simulink subsystem "PieroAJModelz"  (R2023b)
settings: Solver=VariableStepAuto  StartTime=0.0  StopTime=10.0  RelTol=1e-3
settings Model: Creator=Antonio  LastModifiedBy=Antonio

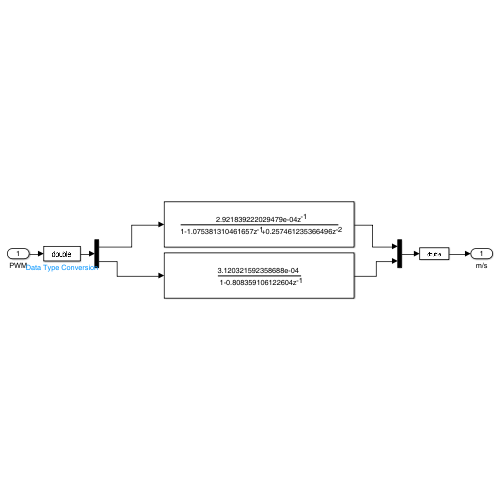
[thumbnail: Simulink's stored preview of the top-level diagram]
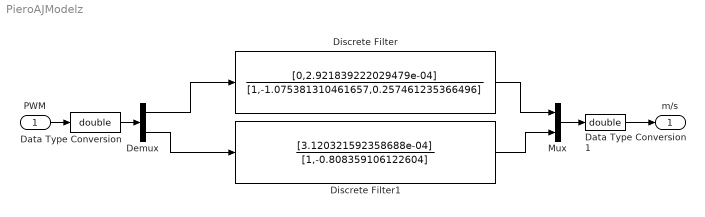
== system PieroAJModelz ==
  PWM : Inport
  Data Type Conversion : DataTypeConversion  OutDataTypeStr=double  SaturateOnIntegerOverflow=off  RndMeth=Floor
  Data Type Conversion1 : DataTypeConversion  OutDataTypeStr=double  SaturateOnIntegerOverflow=off  RndMeth=Floor
  Demux : Demux  Outputs=2
  Discrete Filter : DiscreteFilter  Numerator=[0,2.921839222029479e-04]  Denominator=[1,-1.075381310461657,0.257461235366496]
  Discrete Filter1 : DiscreteFilter  Numerator=[3.120321592358688e-04]  Denominator=[1,-0.808359106122604]
  Mux : Mux  Inputs=2
  m/s : Outport
  wires:
  Demux/1 -> Discrete Filter/1
  Demux/2 -> Discrete Filter1/1
  Discrete Filter/1 -> Mux/1
  Discrete Filter1/1 -> Mux/2
  PWM/1 -> Data Type Conversion/1
  Data Type Conversion/1 -> Demux/1
  Mux/1 -> Data Type Conversion1/1
  Data Type Conversion1/1 -> m/s/1
